simulink model "missing_part"  (R2023b)
settings: Solver=VariableStepAuto  StartTime=0.0  StopTime=10.0  RelTol=1e-3
undefined symbols (not defined in the file): threshold
settings Model: Creator=developer  LastModifiedBy=developer

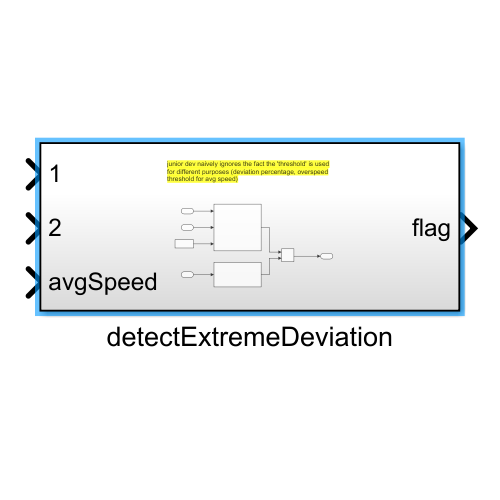
[thumbnail: Simulink's stored preview of the top-level diagram]
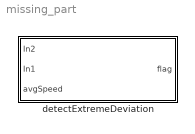
== system missing_part ==
  detectExtremeDeviation : Subsystem

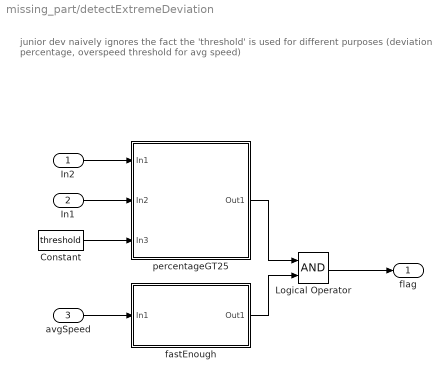
== system missing_part/detectExtremeDeviation ==
  note: junior dev naively ignores the fact the 'threshold' is used for different purposes (deviation percentage, overspeed threshold for avg speed)
  In2 : Inport
  In1 : Inport  Port=2
  avgSpeed : Inport  Port=3
  Constant : Constant  Value=threshold
  Logical Operator : Logic  AllPortsSameDT=off  OutDataTypeStr=boolean
  fastEnough : Subsystem
  percentageGT25 : Subsystem
  flag : Outport
  wires:
  In2/1 -> percentageGT25/1(In1)
  Logical Operator/1 -> flag/1
  In1/1 -> percentageGT25/2(In2)
  Constant/1 -> percentageGT25/3(In3)
  avgSpeed/1 -> fastEnough/1(In1)
  percentageGT25/1(Out1) -> Logical Operator/1
  fastEnough/1(Out1) -> Logical Operator/2

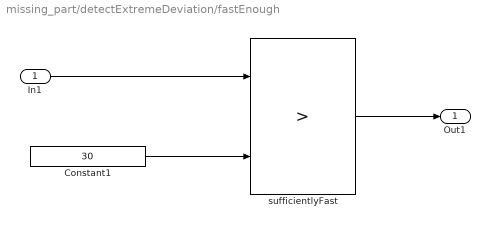
== system missing_part/detectExtremeDeviation/fastEnough ==
  In1 : Inport
  Constant1 : Constant  Value=30
  sufficientlyFast : RelationalOperator  Operator=>  OutDataTypeStr=boolean  RndMeth=Simplest  InputSameDT=off
  Out1 : Outport
  wires:
  Constant1/1 -> sufficientlyFast/2
  In1/1 -> sufficientlyFast/1
  sufficientlyFast/1 -> Out1/1

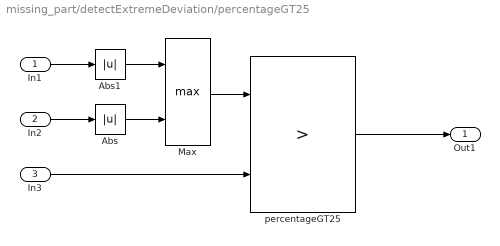
== system missing_part/detectExtremeDeviation/percentageGT25 ==
  In1 : Inport
  In2 : Inport  Port=2
  In3 : Inport  Port=3
  Abs : Abs  SaturateOnIntegerOverflow=off
  Abs1 : Abs  SaturateOnIntegerOverflow=off
  Max : MinMax  Function=max  Inputs=2
  percentageGT25 : RelationalOperator  Operator=>  OutDataTypeStr=boolean  RndMeth=Simplest  InputSameDT=off
  Out1 : Outport
  wires:
  Max/1 -> percentageGT25/1
  Abs1/1 -> Max/1
  percentageGT25/1 -> Out1/1
  In3/1 -> percentageGT25/2
  Abs/1 -> Max/2
  In2/1 -> Abs/1
  In1/1 -> Abs1/1
